simulink model "CAV1553B_PCI_RT_Send"  (Simulink 7.8)
settings: Solver=ode45  StartTime=0.0  StopTime=10.0  RelTol=1e-3
settings Model: Creator=KLJS067  LastModifiedBy=Administrator
settings DebuggingCC: FcnCallInpInsideContextMsg=Use local settings  StrictBusMsg=Warning

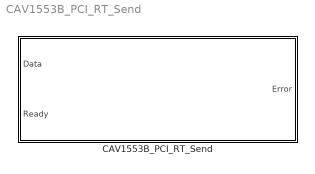
== system CAV1553B_PCI_RT_Send ==
  CAV1553B_PCI_RT_Send : Subsystem  mask(CAV_1553B_PCI RT Send){pci_id=0, chan_id=0, bfirst=1, sourcert_add=0, sourcert_subadd=0}
      mask prompts: pci_id "PCI ID"; chan_id "Channel ID"; bfirst "First Use"; sourcert_add "Remote Terminal"; sourcert_subadd "Sub-Address"
      mask help: This block is used for RT to send messages .
      mask init:
      | displayblock=sprintf('\n1553B RT Send\nPCI Id: %d\nChannel Id: %d\nRT Add: %d\nSub RT: %d\n', pci_id, chan_id,sourcert_add,sourcert_subadd);
      mask StyleString: edit,edit,popup(1|2),edit,edit
      mask CallbackString:
      | ||bfir = get_param(gcb,'bfirst');
      | 
      | if(strcmp(bfir,'1')),
      |     set_param(gcb,'MaskEnables',{'on';'on';'off';'on';'on'}),
      | else
      |     set_param(gcb,'MaskEnables',{'on';'on';'off';'on';'on'}),
      | end
      | ||
      mask Display: disp(displayblock);

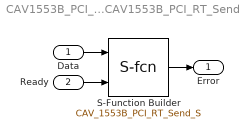
== system CAV1553B_PCI_RT_Send/CAV1553B_PCI_RT_Send ==
  Data : Inport
  Ready : Inport  Port=2
  S-Function Builder : S-Function  InitFcn=try, set_param(gcb,'FunctionName','CAV_1553B_PCI_RT_Send_S'), end  FunctionName=CAV_1553B_PCI_RT_Send_S  Parameters=pci_id,chan_id,bfirst,sourcert_add,sourcert_subadd  WizardData=DataTag0  EnableBusSupport=off  mask(S-Function Builder){}
      mask help: The S-Function Builder block creates a wrapper C-MEX S-function from your supplied C code with multiple input ports, output ports, and a variable number of scalar, vector, or matrix parameters. The input and output ports can propagate Simulink built-in data types, fixed-point datatypes, complex, frame, 1-D, and 2-D signals. This block also supports discrete and continuous states of type real. You can optionally have the block generate a TLC file to be used with Real-Time Workshop for code generation.
      mask init:
      | val = [[.9  0.75 0.75 1 1 .9 .9 1]',[1 1 0.75 0.75 .9 .9 1 .9]'];try , sys = get_param(gcb,'SfunBuilderFcnName');if isempty(sys), sys = get_param(gcb,'FunctionName'); end,catch, sys = get_param(gcb,'FunctionName'); end
      settings: CopyFcn=set_param(gcbh,'LinkStatus','none')  PreSaveFcn=try, set_param(gcb,'FunctionName','CAV_1553B_PCI_RT_Send_S'), end  OpenFcn=sfunctionwizard(gcbh)
      mask Display: plot(val(:,1),val(:,2)),disp(sys)port_label('input',1,'u0')port_label('input',2,'u1')port_label('output',1,'y0')
  Error : Outport
  wires:
  Data/1 -> S-Function Builder/1
  S-Function Builder/1 -> Error/1
  Ready/1 -> S-Function Builder/2
